simulink model "AirCtl_Mon"  (R2016b)
settings: configuration reference "CodeGenConfigSet" (kept outside this file)
values from neighbouring files (symbols this model uses):
  AirCtl_dnEngTrans_C = Calibration.Parameter    [init_AirCtl_Mon.m]    (also in init_AirCtl_Mon_SIL.m = Simulink.Parameter)
  AirCtl_dqLeadTrans_C = Calibration.Parameter    [init_AirCtl_Mon.m]    (also in init_AirCtl_Mon_SIL.m = Simulink.Parameter)
  AirCtl_drAPPTrans_C = Calibration.Parameter    [init_AirCtl_Mon.m]    (also in init_AirCtl_Mon_SIL.m = Simulink.Parameter)
  AirCtl_facActDesVal_C = Calibration.Parameter    [init_AirCtl_Mon.m]    (also in init_AirCtl_Mon_SIL.m = Simulink.Parameter)
  AirCtl_facEngTempSmkHysCor_CUR = Calibration.Parameter    [init_AirCtl_Mon.m]    (also in init_AirCtl_Mon_SIL.m = Simulink.Parameter)
  AirCtl_facEngTempSmkHysCor_CURX = Calibration.Parameter    [init_AirCtl_Mon.m]    (also in init_AirCtl_Mon_SIL.m = Simulink.Parameter)
  AirCtl_facEnvPresSmkHysCor_CUR = Calibration.Parameter    [init_AirCtl_Mon.m]    (also in init_AirCtl_Mon_SIL.m = Simulink.Parameter)
  AirCtl_facEnvPresSmkHysCor_CURX = Calibration.Parameter    [init_AirCtl_Mon.m]    (also in init_AirCtl_Mon_SIL.m = Simulink.Parameter)
  AirCtl_mMaxDvt_MAP = Calibration.Parameter    [init_AirCtl_Mon.m]    (also in init_AirCtl_Mon_SIL.m = Simulink.Parameter)
  AirCtl_mMaxDvt_MAPX = Calibration.Parameter    [init_AirCtl_Mon.m]    (also in init_AirCtl_Mon_SIL.m = Simulink.Parameter)
  AirCtl_mMaxDvt_MAPY = Calibration.Parameter    [init_AirCtl_Mon.m]    (also in init_AirCtl_Mon_SIL.m = Simulink.Parameter)
  AirCtl_mMinDvt_MAP = Calibration.Parameter    [init_AirCtl_Mon.m]    (also in init_AirCtl_Mon_SIL.m = Simulink.Parameter)
  AirCtl_mMinDvt_MAPX = Calibration.Parameter    [init_AirCtl_Mon.m]    (also in init_AirCtl_Mon_SIL.m = Simulink.Parameter)
  AirCtl_mMinDvt_MAPY = Calibration.Parameter    [init_AirCtl_Mon.m]    (also in init_AirCtl_Mon_SIL.m = Simulink.Parameter)
  AirCtl_nLoIdl_C = Calibration.Parameter    [init_AirCtl_Mon.m]    (also in init_AirCtl_Mon_SIL.m = Simulink.Parameter)
  AirCtl_nOvrRun_C = Calibration.Parameter    [init_AirCtl_Mon.m]    (also in init_AirCtl_Mon_SIL.m = Simulink.Parameter)
  AirCtl_numAirTempMon_C = Calibration.Parameter    [init_AirCtl_Mon.m]    (also in init_AirCtl_Mon_SIL.m = Simulink.Parameter)
  AirCtl_numEngTempMon_C = Calibration.Parameter    [init_AirCtl_Mon.m]    (also in init_AirCtl_Mon_SIL.m = Simulink.Parameter)
  AirCtl_pAirHi_C = Calibration.Parameter    [init_AirCtl_Mon.m]    (also in init_AirCtl_Mon_SIL.m = Simulink.Parameter)
  AirCtl_pAirLo_C = Calibration.Parameter    [init_AirCtl_Mon.m]    (also in init_AirCtl_Mon_SIL.m = Simulink.Parameter)
  AirCtl_qEngTempSmkHysCor_MAP = Calibration.Parameter    [init_AirCtl_Mon.m]    (also in init_AirCtl_Mon_SIL.m = Simulink.Parameter)
  AirCtl_qEngTempSmkHysCor_MAPX = Calibration.Parameter    [init_AirCtl_Mon.m]    (also in init_AirCtl_Mon_SIL.m = Simulink.Parameter)
  AirCtl_qEngTempSmkHysCor_MAPY = Calibration.Parameter    [init_AirCtl_Mon.m]    (also in init_AirCtl_Mon_SIL.m = Simulink.Parameter)
  AirCtl_qEnvPresSmkHysCor_MAP = Calibration.Parameter    [init_AirCtl_Mon.m]    (also in init_AirCtl_Mon_SIL.m = Simulink.Parameter)
  AirCtl_qEnvPresSmkHysCor_MAPX = Calibration.Parameter    [init_AirCtl_Mon.m]    (also in init_AirCtl_Mon_SIL.m = Simulink.Parameter)
  AirCtl_qEnvPresSmkHysCor_MAPY = Calibration.Parameter    [init_AirCtl_Mon.m]    (also in init_AirCtl_Mon_SIL.m = Simulink.Parameter)
  AirCtl_qOvrRun_C = Calibration.Parameter    [init_AirCtl_Mon.m]    (also in init_AirCtl_Mon_SIL.m = Simulink.Parameter)
  AirCtl_qSmkHys_MAP = Calibration.Parameter    [init_AirCtl_Mon.m]    (also in init_AirCtl_Mon_SIL.m = Simulink.Parameter)
  AirCtl_qSmkHys_MAPX = Calibration.Parameter    [init_AirCtl_Mon.m]    (also in init_AirCtl_Mon_SIL.m = Simulink.Parameter)
  AirCtl_qSmkHys_MAPY = Calibration.Parameter    [init_AirCtl_Mon.m]    (also in init_AirCtl_Mon_SIL.m = Simulink.Parameter)
  AirCtl_qSwtSmkHi_C = Calibration.Parameter    [init_AirCtl_Mon.m]    (also in init_AirCtl_Mon_SIL.m = Simulink.Parameter)
  AirCtl_qSwtSmkLo_C = Calibration.Parameter    [init_AirCtl_Mon.m]    (also in init_AirCtl_Mon_SIL.m = Simulink.Parameter)
  AirCtl_rEGRDflVal_CA = Calibration.Parameter    [init_AirCtl_Mon.m]    (also in init_AirCtl_Mon_SIL.m = Simulink.Parameter)
  AirCtl_rTVADflVal_CA = Calibration.Parameter    [init_AirCtl_Mon.m]    (also in init_AirCtl_Mon_SIL.m = Simulink.Parameter)
  AirCtl_stPrioMon_CA = Calibration.Parameter    [init_AirCtl_Mon.m]    (also in init_AirCtl_Mon_SIL.m = Simulink.Parameter)
  AirCtl_swtGovDvtMonEna_C = Calibration.Parameter    [init_AirCtl_Mon.m]    (also in init_AirCtl_Mon_SIL.m = Simulink.Parameter)
  AirCtl_tAirCldHi_C = Calibration.Parameter    [init_AirCtl_Mon.m]    (also in init_AirCtl_Mon_SIL.m = Simulink.Parameter)
  AirCtl_tAirCldLo_C = Calibration.Parameter    [init_AirCtl_Mon.m]    (also in init_AirCtl_Mon_SIL.m = Simulink.Parameter)
  AirCtl_tAirWrmHi_C = Calibration.Parameter    [init_AirCtl_Mon.m]    (also in init_AirCtl_Mon_SIL.m = Simulink.Parameter)
  AirCtl_tAirWrmLo_C = Calibration.Parameter    [init_AirCtl_Mon.m]    (also in init_AirCtl_Mon_SIL.m = Simulink.Parameter)
  AirCtl_tClntCldHi_C = Calibration.Parameter    [init_AirCtl_Mon.m]    (also in init_AirCtl_Mon_SIL.m = Simulink.Parameter)
  AirCtl_tClntCldLo_C = Calibration.Parameter    [init_AirCtl_Mon.m]    (also in init_AirCtl_Mon_SIL.m = Simulink.Parameter)
  AirCtl_tClntWrmHi_C = Calibration.Parameter    [init_AirCtl_Mon.m]    (also in init_AirCtl_Mon_SIL.m = Simulink.Parameter)
  AirCtl_tClntWrmLo_C = Calibration.Parameter    [init_AirCtl_Mon.m]    (also in init_AirCtl_Mon_SIL.m = Simulink.Parameter)
  AirCtl_tiCldStrt_CUR = Calibration.Parameter    [init_AirCtl_Mon.m]    (also in init_AirCtl_Mon_SIL.m = Simulink.Parameter)
  AirCtl_tiCldStrt_CURX = Calibration.Parameter    [init_AirCtl_Mon.m]    (also in init_AirCtl_Mon_SIL.m = Simulink.Parameter)
  AirCtl_tiClth_C = Calibration.Parameter    [init_AirCtl_Mon.m]    (also in init_AirCtl_Mon_SIL.m = Simulink.Parameter)
  AirCtl_tiDynSmkDly_C = Calibration.Parameter    [init_AirCtl_Mon.m]    (also in init_AirCtl_Mon_SIL.m = Simulink.Parameter)
  AirCtl_tiGovDvtMaxDebDef_C = Calibration.Parameter    [init_AirCtl_Mon.m]    (also in init_AirCtl_Mon_SIL.m = Simulink.Parameter)
  AirCtl_tiGovDvtMaxDebOk_C = Calibration.Parameter    [init_AirCtl_Mon.m]    (also in init_AirCtl_Mon_SIL.m = Simulink.Parameter)
  AirCtl_tiGovDvtMinDebDef_C = Calibration.Parameter    [init_AirCtl_Mon.m]    (also in init_AirCtl_Mon_SIL.m = Simulink.Parameter)
  AirCtl_tiGovDvtMinDebOk_C = Calibration.Parameter    [init_AirCtl_Mon.m]    (also in init_AirCtl_Mon_SIL.m = Simulink.Parameter)
  AirCtl_tiLoIdl_C = Calibration.Parameter    [init_AirCtl_Mon.m]    (also in init_AirCtl_Mon_SIL.m = Simulink.Parameter)
  AirCtl_tiStatSmkDly_C = Calibration.Parameter    [init_AirCtl_Mon.m]    (also in init_AirCtl_Mon_SIL.m = Simulink.Parameter)
  AirCtl_tiTransDly_C = Calibration.Parameter    [init_AirCtl_Mon.m]    (also in init_AirCtl_Mon_SIL.m = Simulink.Parameter)
  AirCtl_uBattThres_C = Calibration.Parameter    [init_AirCtl_Mon.m]    (also in init_AirCtl_Mon_SIL.m = Simulink.Parameter)
  ASMod_numBnk_C = Calibration.Parameter    [init_AirCtl_Mon.m]    (also in init_AirCtl_Mon_SIL.m = Simulink.Parameter)
  Epm_numCyl_C = Calibration.Parameter    [init_AirCtl_Mon.m]    (also in init_AirCtl_Mon_SIL.m = Simulink.Parameter)
undefined symbols (not defined in the file or in its folder): AirCtl_Mon_DT, EngState_conv, Switch_conv
libraries: simulink x45, CXLib x23
(part 4 of 4)

== system AirCtl_Mon/CheckPrio/If Action Subsystem20 ==
  note: %[1]~[21]%
  Action Port : ActionPort  InitializeStates=reset  ActionType=then
  Constant1 : Constant  Value=22  OutDataTypeStr=uint8
  Constant6 : Constant  Value=AirCtl_stPrioMon_CA
  Selector2 : Selector  IndexMode=Zero-based  InputPortWidth=30  IndexOptions=Index vector (port)  Indices=[1 3]  OutputSizes=1
  priority22 : Outport  OutputWhenDisabled=reset  InitialOutput=0
  wires:
  Constant6/1 -> Selector2/1
  Constant1/1 -> Selector2/2
  Selector2/1 -> priority22/1

== system AirCtl_Mon/CheckPrio/If Action Subsystem21 ==
  note: %[1]~[21]%
  Action Port : ActionPort  InitializeStates=reset  ActionType=then
  Constant1 : Constant  Value=23  OutDataTypeStr=uint8
  Constant6 : Constant  Value=AirCtl_stPrioMon_CA
  Selector2 : Selector  IndexMode=Zero-based  InputPortWidth=30  IndexOptions=Index vector (port)  Indices=[1 3]  OutputSizes=1
  priority23 : Outport  OutputWhenDisabled=reset  InitialOutput=0
  wires:
  Selector2/1 -> priority23/1
  Constant1/1 -> Selector2/2
  Constant6/1 -> Selector2/1

== system AirCtl_Mon/CheckPrio/If Action Subsystem22 ==
  note: %[1]~[21]%
  Action Port : ActionPort  InitializeStates=reset  ActionType=then
  Constant1 : Constant  Value=24  OutDataTypeStr=uint8
  Constant6 : Constant  Value=AirCtl_stPrioMon_CA
  Selector2 : Selector  IndexMode=Zero-based  InputPortWidth=30  IndexOptions=Index vector (port)  Indices=[1 3]  OutputSizes=1
  priority24 : Outport  OutputWhenDisabled=reset  InitialOutput=0
  wires:
  Constant6/1 -> Selector2/1
  Constant1/1 -> Selector2/2
  Selector2/1 -> priority24/1

== system AirCtl_Mon/CheckPrio/If Action Subsystem23 ==
  Action Port : ActionPort  InitializeStates=reset  ActionType=then
  Constant1 : Constant  Value=25  OutDataTypeStr=uint8
  Constant6 : Constant  Value=AirCtl_stPrioMon_CA
  Selector2 : Selector  IndexMode=Zero-based  InputPortWidth=30  IndexOptions=Index vector (port)  Indices=[1 3]  OutputSizes=1
  priority25 : Outport  OutputWhenDisabled=reset  InitialOutput=0
  wires:
  Selector2/1 -> priority25/1
  Constant1/1 -> Selector2/2
  Constant6/1 -> Selector2/1

== system AirCtl_Mon/CheckPrio/If Action Subsystem24 ==
  Action Port : ActionPort  InitializeStates=reset  ActionType=then
  Constant1 : Constant  Value=26  OutDataTypeStr=uint8
  Constant6 : Constant  Value=AirCtl_stPrioMon_CA
  Selector2 : Selector  IndexMode=Zero-based  InputPortWidth=30  IndexOptions=Index vector (port)  Indices=[1 3]  OutputSizes=1
  priority26 : Outport  OutputWhenDisabled=reset  InitialOutput=0
  wires:
  Constant6/1 -> Selector2/1
  Constant1/1 -> Selector2/2
  Selector2/1 -> priority26/1

== system AirCtl_Mon/CheckPrio/If Action Subsystem25 ==
  note: %[1]~[21]%
  Action Port : ActionPort  InitializeStates=reset  ActionType=then
  Constant1 : Constant  Value=19  OutDataTypeStr=uint8
  Constant6 : Constant  Value=AirCtl_stPrioMon_CA
  Selector2 : Selector  IndexMode=Zero-based  InputPortWidth=30  IndexOptions=Index vector (port)  Indices=[1 3]  OutputSizes=1
  priority19 : Outport  OutputWhenDisabled=reset  InitialOutput=0
  wires:
  Selector2/1 -> priority19/1
  Constant1/1 -> Selector2/2
  Constant6/1 -> Selector2/1

== system AirCtl_Mon/CheckPrio/If Action Subsystem26 ==
  Action Port : ActionPort  InitializeStates=reset  ActionType=then
  Constant1 : Constant  Value=27  OutDataTypeStr=uint8
  Constant6 : Constant  Value=AirCtl_stPrioMon_CA
  Selector2 : Selector  IndexMode=Zero-based  InputPortWidth=30  IndexOptions=Index vector (port)  Indices=[1 3]  OutputSizes=1
  priority27 : Outport  OutputWhenDisabled=reset  InitialOutput=0
  wires:
  Selector2/1 -> priority27/1
  Constant1/1 -> Selector2/2
  Constant6/1 -> Selector2/1

== system AirCtl_Mon/CheckPrio/If Action Subsystem27 ==
  Action Port : ActionPort  InitializeStates=reset  ActionType=then
  Constant1 : Constant  Value=28  OutDataTypeStr=uint8
  Constant6 : Constant  Value=AirCtl_stPrioMon_CA
  Selector2 : Selector  IndexMode=Zero-based  InputPortWidth=30  IndexOptions=Index vector (port)  Indices=[1 3]  OutputSizes=1
  priority28 : Outport  OutputWhenDisabled=reset  InitialOutput=0
  wires:
  Constant6/1 -> Selector2/1
  Constant1/1 -> Selector2/2
  Selector2/1 -> priority28/1

== system AirCtl_Mon/CheckPrio/If Action Subsystem28 ==
  Action Port : ActionPort  InitializeStates=reset  ActionType=then
  Constant1 : Constant  Value=29  OutDataTypeStr=uint8
  Constant6 : Constant  Value=AirCtl_stPrioMon_CA
  Selector2 : Selector  IndexMode=Zero-based  InputPortWidth=30  IndexOptions=Index vector (port)  Indices=[1 3]  OutputSizes=1
  priority29 : Outport  OutputWhenDisabled=reset  InitialOutput=0
  wires:
  Selector2/1 -> priority29/1
  Constant1/1 -> Selector2/2
  Constant6/1 -> Selector2/1

== system AirCtl_Mon/CheckPrio/If Action Subsystem3 ==
  note: %[1]~[21]%
  Action Port : ActionPort  InitializeStates=reset  ActionType=then
  Constant1 : Constant  Value=4  OutDataTypeStr=uint8
  Constant6 : Constant  Value=AirCtl_stPrioMon_CA
  Selector2 : Selector  IndexMode=Zero-based  InputPortWidth=30  IndexOptions=Index vector (port)  Indices=[1 3]  OutputSizes=1
  priority4 : Outport  OutputWhenDisabled=reset  InitialOutput=0
  wires:
  Constant6/1 -> Selector2/1
  Constant1/1 -> Selector2/2
  Selector2/1 -> priority4/1

== system AirCtl_Mon/CheckPrio/If Action Subsystem4 ==
  note: %[1]~[21]%
  Action Port : ActionPort  InitializeStates=reset  ActionType=then
  Constant1 : Constant  Value=5  OutDataTypeStr=uint8
  Constant6 : Constant  Value=AirCtl_stPrioMon_CA
  Selector2 : Selector  IndexMode=Zero-based  InputPortWidth=30  IndexOptions=Index vector (port)  Indices=[1 3]  OutputSizes=1
  priority5 : Outport  OutputWhenDisabled=reset  InitialOutput=0
  wires:
  Selector2/1 -> priority5/1
  Constant1/1 -> Selector2/2
  Constant6/1 -> Selector2/1

== system AirCtl_Mon/CheckPrio/If Action Subsystem5 ==
  note: %[1]~[21]%
  Action Port : ActionPort  InitializeStates=reset  ActionType=then
  Constant1 : Constant  Value=6  OutDataTypeStr=uint8
  Constant6 : Constant  Value=AirCtl_stPrioMon_CA
  Selector2 : Selector  IndexMode=Zero-based  InputPortWidth=30  IndexOptions=Index vector (port)  Indices=[1 3]  OutputSizes=1
  priority6 : Outport  OutputWhenDisabled=reset  InitialOutput=0
  wires:
  Constant6/1 -> Selector2/1
  Constant1/1 -> Selector2/2
  Selector2/1 -> priority6/1

== system AirCtl_Mon/CheckPrio/If Action Subsystem6 ==
  note: %[1]~[21]%
  Action Port : ActionPort  InitializeStates=reset  ActionType=then
  Constant1 : Constant  Value=7  OutDataTypeStr=uint8
  Constant6 : Constant  Value=AirCtl_stPrioMon_CA
  Selector2 : Selector  IndexMode=Zero-based  InputPortWidth=30  IndexOptions=Index vector (port)  Indices=[1 3]  OutputSizes=1
  priority7 : Outport  OutputWhenDisabled=reset  InitialOutput=0
  wires:
  Selector2/1 -> priority7/1
  Constant1/1 -> Selector2/2
  Constant6/1 -> Selector2/1

== system AirCtl_Mon/CheckPrio/If Action Subsystem7 ==
  note: %[1]~[21]%
  Action Port : ActionPort  InitializeStates=reset  ActionType=then
  Constant1 : Constant  Value=8  OutDataTypeStr=uint8
  Constant6 : Constant  Value=AirCtl_stPrioMon_CA
  Selector2 : Selector  IndexMode=Zero-based  InputPortWidth=30  IndexOptions=Index vector (port)  Indices=[1 3]  OutputSizes=1
  priority8 : Outport  OutputWhenDisabled=reset  InitialOutput=0
  wires:
  Constant6/1 -> Selector2/1
  Constant1/1 -> Selector2/2
  Selector2/1 -> priority8/1

== system AirCtl_Mon/CheckPrio/If Action Subsystem8 ==
  note: %[1]~[21]%
  Action Port : ActionPort  InitializeStates=reset  ActionType=then
  Constant1 : Constant  Value=9  OutDataTypeStr=uint8
  Constant6 : Constant  Value=AirCtl_stPrioMon_CA
  Selector2 : Selector  IndexMode=Zero-based  InputPortWidth=30  IndexOptions=Index vector (port)  Indices=[1 3]  OutputSizes=1
  priority9 : Outport  OutputWhenDisabled=reset  InitialOutput=0
  wires:
  Selector2/1 -> priority9/1
  Constant1/1 -> Selector2/2
  Constant6/1 -> Selector2/1

== system AirCtl_Mon/CheckPrio/If Action Subsystem9 ==
  note: %[1]~[21]%
  Action Port : ActionPort  InitializeStates=reset  ActionType=then
  Constant1 : Constant  Value=10  OutDataTypeStr=uint8
  Constant6 : Constant  Value=AirCtl_stPrioMon_CA
  Selector2 : Selector  IndexMode=Zero-based  InputPortWidth=30  IndexOptions=Index vector (port)  Indices=[1 3]  OutputSizes=1
  priority10 : Outport  OutputWhenDisabled=reset  InitialOutput=0
  wires:
  Constant6/1 -> Selector2/1
  Constant1/1 -> Selector2/2
  Selector2/1 -> priority10/1

== system AirCtl_Mon/EngTemp and CldStrtMon/Sample and Hold ==
  In1 : Inport
  Trigger : TriggerPort  VariantControl=Variant  ZeroCross=off
  Out1 : Outport  InitialOutput=0
  wires:
  In1/1 -> Out1/1

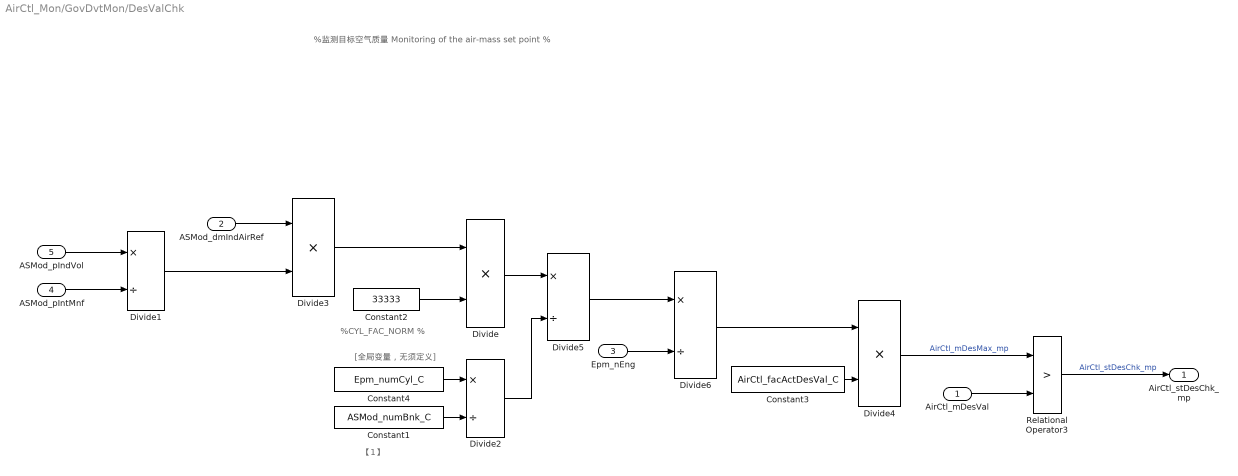
== system AirCtl_Mon/GovDvtMon/DesValChk ==
  note: %监测目标空气质量
      | Monitoring of the air-mass set point %
  note: %CYL_FAC_NORM %
  note: [全局变量，无须定义]
  note: 【1】
  AirCtl_mDesVal : Inport
  ASMod_dmIndAirRef : Inport  Port=2
  Epm_nEng : Inport  Port=3
  ASMod_pIntMnf : Inport  Port=4
  ASMod_pIndVol : Inport  Port=5
  Constant1 : Constant  Value=ASMod_numBnk_C
  Constant2 : Constant  Value=33333  OutDataTypeStr=uint16
  Constant3 : Constant  Value=AirCtl_facActDesVal_C
  Constant4 : Constant  Value=Epm_numCyl_C
  Divide : Product  Inputs=**  SaturateOnIntegerOverflow=on
  Divide1 : Product  Inputs=*/  OutDataTypeStr=Prc_Fact100  SaturateOnIntegerOverflow=on
  Divide2 : Product  Inputs=*/  OutDataTypeStr=uint8  SaturateOnIntegerOverflow=on
  Divide3 : Product  Inputs=**  OutDataTypeStr=AirMassPerTime  SaturateOnIntegerOverflow=on
  Divide4 : Product  Inputs=**  OutDataTypeStr=AirMass_mg_hub  SaturateOnIntegerOverflow=on
  Divide5 : Product  Inputs=*/  SaturateOnIntegerOverflow=on
  Divide6 : Product  Inputs=*/  OutDataTypeStr=AirMass_mg_hub  SaturateOnIntegerOverflow=on
  Relational Operator3 : RelationalOperator  Operator=>  OutDataTypeStr=boolean  RndMeth=Simplest  InputSameDT=on
  AirCtl_stDesChk_mp : Outport
  wires:
  ASMod_pIndVol/1 -> Divide1/1
  ASMod_pIntMnf/1 -> Divide1/2
  Divide6/1 -> Divide4/1
  Divide5/1 -> Divide6/1
  Divide3/1 -> Divide/1
  Divide1/1 -> Divide3/2
  Divide/1 -> Divide5/1
  Constant2/1 -> Divide/2
  Relational Operator3/1 -> AirCtl_stDesChk_mp/1  "AirCtl_stDesChk_mp"
  AirCtl_mDesVal/1 -> Relational Operator3/2
  Divide4/1 -> Relational Operator3/1  "AirCtl_mDesMax_mp"
  Constant3/1 -> Divide4/2
  Epm_nEng/1 -> Divide6/2
  Divide2/1 -> Divide5/2
  Constant4/1 -> Divide2/1
  Constant1/1 -> Divide2/2
  ASMod_dmIndAirRef/1 -> Divide3/1

== system AirCtl_Mon/GovDvtMon/VarDebSetDFC_inl6 ==
  note: %长期控制偏差故障处理
      | Error debouncing%
  stDebDef : Inport
  stMaxDvt : Inport  Port=2
  stMinDvt : Inport  Port=3
  If5 : If  RequirementInfo={} %GIDa_97b2bc00_94fb_4cdc_b38d_4c9258bbcc9a  IfExpression=u1 ~= 0  ShowElse=off
  MaxHeal1 : Subsystem  TreatAsAtomicUnit=on
  AirCtl_bGovDvtMax_DSM : Outport  Description=DFC of AirCtl_bGovDvtMax  OutMin=0  OutMax=1
  AirCtl_bGovDvtMin_DSM : Outport  Description=DFC of AirCtl_bGovDvtMin  Port=2  OutMin=0  OutMax=1
  wires:
  stMinDvt/1 -> MaxHeal1/2(stMinDvt)
  stMaxDvt/1 -> MaxHeal1/1(stMaxDvt)
  stDebDef/1 -> If5/1
  If5/1 -> MaxHeal1/Action
  MaxHeal1/1(AirCtl_bGovDvtMax_DSM) -> AirCtl_bGovDvtMax_DSM/1
  MaxHeal1/2(AirCtl_bGovDvtMin_DSM) -> AirCtl_bGovDvtMin_DSM/1

== system AirCtl_Mon/GovDvtMon/VarGovDvtLim_inl4 ==
  note: %控制偏差监测限值
      | Limits for monitoring of the control deviation %
  Epm_nEng : Inport
  AirCtl_qMon : Inport  Port=2
  AirCtl_mMaxDvt_MAP : Lookup_n-D  BreakpointsForDimension1=AirCtl_mMaxDvt_MAPY  BreakpointsForDimension2=AirCtl_mMaxDvt_MAPX  BeginIndexSearchUsingPreviousIndexResult=on  Table=AirCtl_mMaxDvt_MAP  TableDataTypeStr=Inherit: Inherit from 'Table data'  ExtrapMethod=Clip  UseLastTableValue=on  InternalRulePriority=Speed  OutDataTypeStr=Inherit: Inherit from 'Table data'  RndMeth=Simplest  SaturateOnIntegerOverflow=on
  AirCtl_mMinDvt_MAP : Lookup_n-D  BreakpointsForDimension1=AirCtl_mMinDvt_MAPY  BreakpointsForDimension2=AirCtl_mMinDvt_MAPX  BeginIndexSearchUsingPreviousIndexResult=on  Table=AirCtl_mMinDvt_MAP  TableDataTypeStr=Inherit: Inherit from 'Table data'  ExtrapMethod=Clip  UseLastTableValue=on  InternalRulePriority=Speed  OutDataTypeStr=Inherit: Inherit from 'Table data'  RndMeth=Simplest  SaturateOnIntegerOverflow=on
  AirCtl_mMaxDvt : Outport
  AirCtl_mMinDvt : Outport  Port=2
  wires:
  AirCtl_mMaxDvt_MAP/1 -> AirCtl_mMaxDvt/1  "AirCtl_mMaxDvt"
  AirCtl_mMinDvt_MAP/1 -> AirCtl_mMinDvt/1  "AirCtl_mMinDvt"
  Epm_nEng/1 -> AirCtl_mMaxDvt_MAP/2, AirCtl_mMinDvt_MAP/2
  AirCtl_qMon/1 -> AirCtl_mMaxDvt_MAP/1, AirCtl_mMinDvt_MAP/1

== system AirCtl_Mon/GovDvtMon/VarGovDvtMonEna_inl8 ==
  note: %激活控制偏差监测
      | Activation of monitoring for a permanent control deviation %
  Constant1 : Constant  Value=Switch_conv.ON  SampleTime=-1
  Constant6 : Constant  Value=AirCtl_swtGovDvtMonEna_C  SampleTime=-1
  Relational Operator3 : RelationalOperator  Operator===  OutDataTypeStr=boolean  RndMeth=Simplest  InputSameDT=on
  AirCtl_stGovDvtMonEna_mp : Outport
  wires:
  Constant6/1 -> Relational Operator3/1
  Constant1/1 -> Relational Operator3/2
  Relational Operator3/1 -> AirCtl_stGovDvtMonEna_mp/1  "AirCtl_stGovDvtMonEna_mp"

== system AirCtl_Mon/SysMon/GetBit2 ==
  u : Inport  OutDataTypeStr=uint8
  bit : Inport  Port=2
  GetBit : Stateflow chart  TreatAsAtomicUnit=on
  dataLength : Constant  Value=dataLength  OutDataTypeStr=uint8
  y : Outport  OutDataTypeStr=boolean
  wires:
  bit/1 -> GetBit/2(BitPos)
  u/1 -> GetBit/1(Value)
  GetBit/1(BitValue) -> y/1
  dataLength/1 -> GetBit/3(data_length)

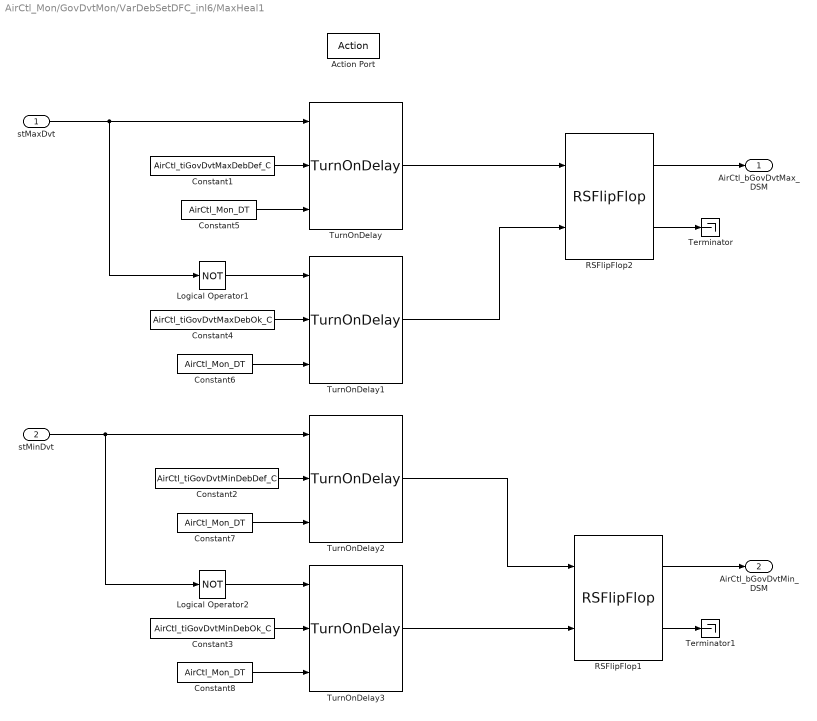
== system AirCtl_Mon/GovDvtMon/VarDebSetDFC_inl6/MaxHeal1 ==
  stMaxDvt : Inport
  stMinDvt : Inport  Port=2
  Action Port : ActionPort  ActionType=then
  Constant1 : Constant  Value=AirCtl_tiGovDvtMaxDebDef_C  SampleTime=-1
  Constant2 : Constant  Value=AirCtl_tiGovDvtMinDebDef_C  SampleTime=-1
  Constant3 : Constant  Value=AirCtl_tiGovDvtMinDebOk_C  SampleTime=-1
  Constant4 : Constant  Value=AirCtl_tiGovDvtMaxDebOk_C  SampleTime=-1
  Constant{5..8} (4 alike) : Constant  Value=AirCtl_Mon_DT  SampleTime=-1
  Logical Operator1 : Logic  RequirementInfo={} %GIDa_136db9b7_7509_4cd4_8a9c_ea0cc66abd7e  Operator=NOT  AllPortsSameDT=off  OutDataTypeStr=boolean
  Logical Operator2 : Logic  RequirementInfo={} %GIDa_3ac86330_b471_435b_b3df_ea9ba73428cf  Operator=NOT  AllPortsSameDT=off  OutDataTypeStr=boolean
  RSFlipFlop1 : CXLib/RSFlipFlop
  RSFlipFlop2 : CXLib/RSFlipFlop
  Terminator : Terminator
  Terminator1 : Terminator
  TurnOnDelay{,1..3} (4 alike) : CXLib/TurnOnDelay
  AirCtl_bGovDvtMax_DSM : Outport  Description=DFC of AirCtl_bGovDvtMax  OutMin=0  OutMax=1
  AirCtl_bGovDvtMin_DSM : Outport  Description=DFC of AirCtl_bGovDvtMin  Port=2  OutMin=0  OutMax=1
  wires:
  Constant6/1 -> TurnOnDelay1/3
  Constant5/1 -> TurnOnDelay/3
  Constant8/1 -> TurnOnDelay3/3
  Constant7/1 -> TurnOnDelay2/3
  Constant4/1 -> TurnOnDelay1/2
  Constant2/1 -> TurnOnDelay2/2
  stMinDvt/1 -> TurnOnDelay2/1, Logical Operator2/1
  TurnOnDelay3/1 -> RSFlipFlop1/2
  TurnOnDelay2/1 -> RSFlipFlop1/1
  Logical Operator2/1 -> TurnOnDelay3/1
  Constant3/1 -> TurnOnDelay3/2
  Constant1/1 -> TurnOnDelay/2
  stMaxDvt/1 -> TurnOnDelay/1, Logical Operator1/1
  TurnOnDelay1/1 -> RSFlipFlop2/2
  TurnOnDelay/1 -> RSFlipFlop2/1
  Logical Operator1/1 -> TurnOnDelay1/1
  RSFlipFlop2/1 -> AirCtl_bGovDvtMax_DSM/1
  RSFlipFlop2/2 -> Terminator/1
  RSFlipFlop1/1 -> AirCtl_bGovDvtMin_DSM/1
  RSFlipFlop1/2 -> Terminator1/1

== stateflow chart AirCtl_Mon/SysMon/GetBit2/GetBit ==
  (default) -> (junction 2)
  (junction 2) -> (junction 1) [order 1] : [BitPos < data_length]
  (junction 2) -> (junction 8) [order 2] : {BitValue = 0;}
  (junction 1) -> (junction 3) : {BitValue = (Value>>BitPos)&1;}
  (junction 3) -> (junction 8)
  (junction 8) -> (junction 6)
  data: Value input; BitPos input uint8; data_length input uint8; BitValue output boolean

== stateflow chart AirCtl_Mon/CheckPrio/GetBit29/GetBit ==
  (default) -> (junction 2)
  (junction 2) -> (junction 1) [order 1] : [BitPos < data_length]
  (junction 2) -> (junction 8) [order 2] : {BitValue = 0;}
  (junction 1) -> (junction 3) : {BitValue = (Value>>BitPos)&1;}
  (junction 3) -> (junction 8)
  (junction 8) -> (junction 6)
  data: Value input; BitPos input uint8; data_length input uint8; BitValue output boolean

== stateflow chart AirCtl_Mon/CheckPrio/GetBit1/GetBit ==
  (default) -> (junction 2)
  (junction 2) -> (junction 1) [order 1] : [BitPos < data_length]
  (junction 2) -> (junction 8) [order 2] : {BitValue = 0;}
  (junction 1) -> (junction 3) : {BitValue = (Value>>BitPos)&1;}
  (junction 3) -> (junction 8)
  (junction 8) -> (junction 6)
  data: Value input; BitPos input uint8; data_length input uint8; BitValue output boolean

== stateflow chart AirCtl_Mon/CheckPrio/GetBit2/GetBit ==
  (default) -> (junction 2)
  (junction 2) -> (junction 1) [order 1] : [BitPos < data_length]
  (junction 2) -> (junction 8) [order 2] : {BitValue = 0;}
  (junction 1) -> (junction 3) : {BitValue = (Value>>BitPos)&1;}
  (junction 3) -> (junction 8)
  (junction 8) -> (junction 6)
  data: Value input; BitPos input uint8; data_length input uint8; BitValue output boolean

== stateflow chart AirCtl_Mon/CheckPrio/GetBit3/GetBit ==
  (default) -> (junction 2)
  (junction 2) -> (junction 1) [order 1] : [BitPos < data_length]
  (junction 2) -> (junction 8) [order 2] : {BitValue = 0;}
  (junction 1) -> (junction 3) : {BitValue = (Value>>BitPos)&1;}
  (junction 3) -> (junction 8)
  (junction 8) -> (junction 6)
  data: Value input; BitPos input uint8; data_length input uint8; BitValue output boolean

== stateflow chart AirCtl_Mon/CheckPrio/GetBit4/GetBit ==
  (default) -> (junction 2)
  (junction 2) -> (junction 1) [order 1] : [BitPos < data_length]
  (junction 2) -> (junction 8) [order 2] : {BitValue = 0;}
  (junction 1) -> (junction 3) : {BitValue = (Value>>BitPos)&1;}
  (junction 3) -> (junction 8)
  (junction 8) -> (junction 6)
  data: Value input; BitPos input uint8; data_length input uint8; BitValue output boolean

== stateflow chart AirCtl_Mon/CheckPrio/GetBit5/GetBit ==
  (default) -> (junction 2)
  (junction 2) -> (junction 1) [order 1] : [BitPos < data_length]
  (junction 2) -> (junction 8) [order 2] : {BitValue = 0;}
  (junction 1) -> (junction 3) : {BitValue = (Value>>BitPos)&1;}
  (junction 3) -> (junction 8)
  (junction 8) -> (junction 6)
  data: Value input; BitPos input uint8; data_length input uint8; BitValue output boolean

== stateflow chart AirCtl_Mon/CheckPrio/GetBit6/GetBit ==
  (default) -> (junction 2)
  (junction 2) -> (junction 1) [order 1] : [BitPos < data_length]
  (junction 2) -> (junction 8) [order 2] : {BitValue = 0;}
  (junction 1) -> (junction 3) : {BitValue = (Value>>BitPos)&1;}
  (junction 3) -> (junction 8)
  (junction 8) -> (junction 6)
  data: Value input; BitPos input uint8; data_length input uint8; BitValue output boolean

== stateflow chart AirCtl_Mon/CheckPrio/GetBit7/GetBit ==
  (default) -> (junction 2)
  (junction 2) -> (junction 1) [order 1] : [BitPos < data_length]
  (junction 2) -> (junction 8) [order 2] : {BitValue = 0;}
  (junction 1) -> (junction 3) : {BitValue = (Value>>BitPos)&1;}
  (junction 3) -> (junction 8)
  (junction 8) -> (junction 6)
  data: Value input; BitPos input uint8; data_length input uint8; BitValue output boolean

== stateflow chart AirCtl_Mon/CheckPrio/GetBit8/GetBit ==
  (default) -> (junction 2)
  (junction 2) -> (junction 1) [order 1] : [BitPos < data_length]
  (junction 2) -> (junction 8) [order 2] : {BitValue = 0;}
  (junction 1) -> (junction 3) : {BitValue = (Value>>BitPos)&1;}
  (junction 3) -> (junction 8)
  (junction 8) -> (junction 6)
  data: Value input; BitPos input uint8; data_length input uint8; BitValue output boolean

== stateflow chart AirCtl_Mon/CheckPrio/GetBit9/GetBit ==
  (default) -> (junction 2)
  (junction 2) -> (junction 1) [order 1] : [BitPos < data_length]
  (junction 2) -> (junction 8) [order 2] : {BitValue = 0;}
  (junction 1) -> (junction 3) : {BitValue = (Value>>BitPos)&1;}
  (junction 3) -> (junction 8)
  (junction 8) -> (junction 6)
  data: Value input; BitPos input uint8; data_length input uint8; BitValue output boolean

== stateflow chart AirCtl_Mon/CheckPrio/GetBit10/GetBit ==
  (default) -> (junction 2)
  (junction 2) -> (junction 1) [order 1] : [BitPos < data_length]
  (junction 2) -> (junction 8) [order 2] : {BitValue = 0;}
  (junction 1) -> (junction 3) : {BitValue = (Value>>BitPos)&1;}
  (junction 3) -> (junction 8)
  (junction 8) -> (junction 6)
  data: Value input; BitPos input uint8; data_length input uint8; BitValue output boolean

== stateflow chart AirCtl_Mon/CheckPrio/GetBit11/GetBit ==
  (default) -> (junction 2)
  (junction 2) -> (junction 1) [order 1] : [BitPos < data_length]
  (junction 2) -> (junction 8) [order 2] : {BitValue = 0;}
  (junction 1) -> (junction 3) : {BitValue = (Value>>BitPos)&1;}
  (junction 3) -> (junction 8)
  (junction 8) -> (junction 6)
  data: Value input; BitPos input uint8; data_length input uint8; BitValue output boolean

== stateflow chart AirCtl_Mon/CheckPrio/GetBit12/GetBit ==
  (default) -> (junction 2)
  (junction 2) -> (junction 1) [order 1] : [BitPos < data_length]
  (junction 2) -> (junction 8) [order 2] : {BitValue = 0;}
  (junction 1) -> (junction 3) : {BitValue = (Value>>BitPos)&1;}
  (junction 3) -> (junction 8)
  (junction 8) -> (junction 6)
  data: Value input; BitPos input uint8; data_length input uint8; BitValue output boolean

== stateflow chart AirCtl_Mon/CheckPrio/GetBit13/GetBit ==
  (default) -> (junction 2)
  (junction 2) -> (junction 1) [order 1] : [BitPos < data_length]
  (junction 2) -> (junction 8) [order 2] : {BitValue = 0;}
  (junction 1) -> (junction 3) : {BitValue = (Value>>BitPos)&1;}
  (junction 3) -> (junction 8)
  (junction 8) -> (junction 6)
  data: Value input; BitPos input uint8; data_length input uint8; BitValue output boolean

== stateflow chart AirCtl_Mon/CheckPrio/GetBit14/GetBit ==
  (default) -> (junction 2)
  (junction 2) -> (junction 1) [order 1] : [BitPos < data_length]
  (junction 2) -> (junction 8) [order 2] : {BitValue = 0;}
  (junction 1) -> (junction 3) : {BitValue = (Value>>BitPos)&1;}
  (junction 3) -> (junction 8)
  (junction 8) -> (junction 6)
  data: Value input; BitPos input uint8; data_length input uint8; BitValue output boolean

== stateflow chart AirCtl_Mon/CheckPrio/GetBit15/GetBit ==
  (default) -> (junction 2)
  (junction 2) -> (junction 1) [order 1] : [BitPos < data_length]
  (junction 2) -> (junction 8) [order 2] : {BitValue = 0;}
  (junction 1) -> (junction 3) : {BitValue = (Value>>BitPos)&1;}
  (junction 3) -> (junction 8)
  (junction 8) -> (junction 6)
  data: Value input; BitPos input uint8; data_length input uint8; BitValue output boolean

== stateflow chart AirCtl_Mon/CheckPrio/GetBit16/GetBit ==
  (default) -> (junction 2)
  (junction 2) -> (junction 1) [order 1] : [BitPos < data_length]
  (junction 2) -> (junction 8) [order 2] : {BitValue = 0;}
  (junction 1) -> (junction 3) : {BitValue = (Value>>BitPos)&1;}
  (junction 3) -> (junction 8)
  (junction 8) -> (junction 6)
  data: Value input; BitPos input uint8; data_length input uint8; BitValue output boolean

== stateflow chart AirCtl_Mon/CheckPrio/GetBit17/GetBit ==
  (default) -> (junction 2)
  (junction 2) -> (junction 1) [order 1] : [BitPos < data_length]
  (junction 2) -> (junction 8) [order 2] : {BitValue = 0;}
  (junction 1) -> (junction 3) : {BitValue = (Value>>BitPos)&1;}
  (junction 3) -> (junction 8)
  (junction 8) -> (junction 6)
  data: Value input; BitPos input uint8; data_length input uint8; BitValue output boolean

== stateflow chart AirCtl_Mon/CheckPrio/GetBit18/GetBit ==
  (default) -> (junction 2)
  (junction 2) -> (junction 1) [order 1] : [BitPos < data_length]
  (junction 2) -> (junction 8) [order 2] : {BitValue = 0;}
  (junction 1) -> (junction 3) : {BitValue = (Value>>BitPos)&1;}
  (junction 3) -> (junction 8)
  (junction 8) -> (junction 6)
  data: Value input; BitPos input uint8; data_length input uint8; BitValue output boolean

== stateflow chart AirCtl_Mon/CheckPrio/GetBit19/GetBit ==
  (default) -> (junction 2)
  (junction 2) -> (junction 1) [order 1] : [BitPos < data_length]
  (junction 2) -> (junction 8) [order 2] : {BitValue = 0;}
  (junction 1) -> (junction 3) : {BitValue = (Value>>BitPos)&1;}
  (junction 3) -> (junction 8)
  (junction 8) -> (junction 6)
  data: Value input; BitPos input uint8; data_length input uint8; BitValue output boolean

== stateflow chart AirCtl_Mon/CheckPrio/GetBit20/GetBit ==
  (default) -> (junction 2)
  (junction 2) -> (junction 1) [order 1] : [BitPos < data_length]
  (junction 2) -> (junction 8) [order 2] : {BitValue = 0;}
  (junction 1) -> (junction 3) : {BitValue = (Value>>BitPos)&1;}
  (junction 3) -> (junction 8)
  (junction 8) -> (junction 6)
  data: Value input; BitPos input uint8; data_length input uint8; BitValue output boolean

== stateflow chart AirCtl_Mon/CheckPrio/GetBit21/GetBit ==
  (default) -> (junction 2)
  (junction 2) -> (junction 1) [order 1] : [BitPos < data_length]
  (junction 2) -> (junction 8) [order 2] : {BitValue = 0;}
  (junction 1) -> (junction 3) : {BitValue = (Value>>BitPos)&1;}
  (junction 3) -> (junction 8)
  (junction 8) -> (junction 6)
  data: Value input; BitPos input uint8; data_length input uint8; BitValue output boolean

== stateflow chart AirCtl_Mon/CheckPrio/GetBit22/GetBit ==
  (default) -> (junction 2)
  (junction 2) -> (junction 1) [order 1] : [BitPos < data_length]
  (junction 2) -> (junction 8) [order 2] : {BitValue = 0;}
  (junction 1) -> (junction 3) : {BitValue = (Value>>BitPos)&1;}
  (junction 3) -> (junction 8)
  (junction 8) -> (junction 6)
  data: Value input; BitPos input uint8; data_length input uint8; BitValue output boolean

== stateflow chart AirCtl_Mon/CheckPrio/GetBit23/GetBit ==
  (default) -> (junction 2)
  (junction 2) -> (junction 1) [order 1] : [BitPos < data_length]
  (junction 2) -> (junction 8) [order 2] : {BitValue = 0;}
  (junction 1) -> (junction 3) : {BitValue = (Value>>BitPos)&1;}
  (junction 3) -> (junction 8)
  (junction 8) -> (junction 6)
  data: Value input; BitPos input uint8; data_length input uint8; BitValue output boolean

== stateflow chart AirCtl_Mon/CheckPrio/GetBit24/GetBit ==
  (default) -> (junction 2)
  (junction 2) -> (junction 1) [order 1] : [BitPos < data_length]
  (junction 2) -> (junction 8) [order 2] : {BitValue = 0;}
  (junction 1) -> (junction 3) : {BitValue = (Value>>BitPos)&1;}
  (junction 3) -> (junction 8)
  (junction 8) -> (junction 6)
  data: Value input; BitPos input uint8; data_length input uint8; BitValue output boolean

== stateflow chart AirCtl_Mon/CheckPrio/GetBit25/GetBit ==
  (default) -> (junction 2)
  (junction 2) -> (junction 1) [order 1] : [BitPos < data_length]
  (junction 2) -> (junction 8) [order 2] : {BitValue = 0;}
  (junction 1) -> (junction 3) : {BitValue = (Value>>BitPos)&1;}
  (junction 3) -> (junction 8)
  (junction 8) -> (junction 6)
  data: Value input; BitPos input uint8; data_length input uint8; BitValue output boolean

== stateflow chart AirCtl_Mon/CheckPrio/GetBit26/GetBit ==
  (default) -> (junction 2)
  (junction 2) -> (junction 1) [order 1] : [BitPos < data_length]
  (junction 2) -> (junction 8) [order 2] : {BitValue = 0;}
  (junction 1) -> (junction 3) : {BitValue = (Value>>BitPos)&1;}
  (junction 3) -> (junction 8)
  (junction 8) -> (junction 6)
  data: Value input; BitPos input uint8; data_length input uint8; BitValue output boolean
